simulink model "Switched_Reluctance_Motor_12bar8_config"  (R2021a)
settings: Solver=VariableStepAuto  StartTime=0.0  StopTime=1  FixedStep=1  MaxStep=1e-6  RelTol=1e-6
values from neighbouring files (symbols this model uses):
  angleArray = [0 0.5 1 1.5 2 2.5 3 3.5 4 4.5 5 5.5 ... (720 elements, 720x1)]    [matlab.mat]
  currentArray = [0 0.5 1 1.5 2 2.5 3 3.5 4 4.5 5 5.5 ... (51 elements, 51x1)]    [matlab.mat]
  fluxdiv = [0 4.83333e-05 9.66666e-05 0.000145 0.000193333 0.000241667 0.00029 0.000338333 0.000386666 0.000435 0.000483333 0.000531666 ... (720 elements, 720x1)]    [matlab.mat]
undefined symbols (not defined in the file or in its folder): iLUT, torqueMatrix
libraries: simulink x3, hdlsllib x1
settings Model: Creator=ADMIN  LastModifiedBy=Anirudh Chidambaram
settings SolverCC: AlgebraicLoopSolver=LineSearch
settings DataIOCC: SaveState=on
settings OptimizationCC: DefaultParameterBehavior=Inlined  EnhancedBackFolding=on  PassReuseOutputArgsAs=Individual arguments  ZeroExternalMemoryAtStartup=off  ZeroInternalMemoryAtStartup=off  OptimizeBlockOrder=speed  DifferentSizesBufferReuse=on  OptimizationCustomize=off  EfficientTunableParamExpr=on
settings DebuggingCC: AlgebraicLoopMsg=none  ParameterOverflowMsg=warning  ParameterTunabilityLossMsg=error  SFMachineParentedDataDiag=warning
settings SFSimCC: MATLABDynamicMemAlloc=off
settings RTWCC: SystemTargetFile=ert.tlc  TemplateMakefile=ert_default_tmf
settings CodeAppCC: ForceParamTrailComments=on  IgnoreCustomStorageClasses=off  OperatorAnnotations=on  SimulinkDataObjDesc=on  SFDataObjDesc=on  InsertBlockDesc=on
settings ERTTargetCC: TargetLangStandard=C99 (ISO)  GenerateSampleERTMain=on  InlinedParameterPlacement=NonHierarchical  ERTCustomFileTemplate=example_file_process.tlc

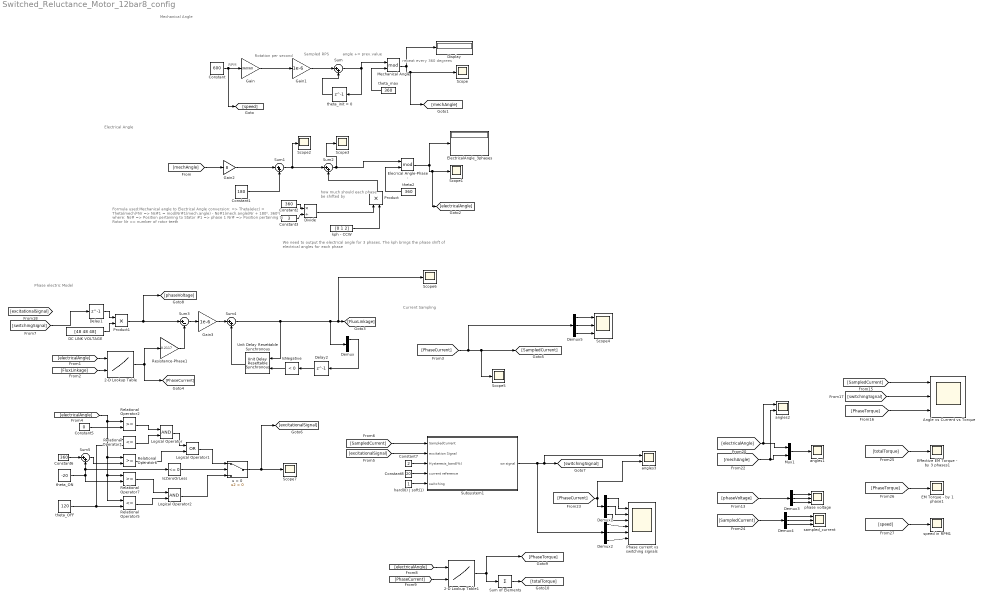
== system Switched_Reluctance_Motor_12bar8_config ==
  note: how much should each phase be shifted by
  note: repeat every 360 degrees
  note: angle += prev.value
  note: Sampled RPS
  note: Rotation per second
  note: RPM
  note: Electrical Angle
  note: Mechanical Angle
  note: Current Sampling
  note: Phase electric Model
  note: We need to output the electrical angle for 3 phases,
      | The kph brings the phase shift of electrical angles for each phase
  note: Formula used:Mechanical angle to Electrical Angle conversion:
      | => Theta(elec) = Theta(mech)*Nr
      |
      | => Ns#1 = mod(Nr#1(mech.angle) - Ns#1(mech.angle)Nr + 180⁰, 360⁰)
      | where:
      | Ns# => Position pertaining to Stator
      | #1	 => phase 1
      | Nr# => Position pertaining to Rotor
      | Nr	 => number of rotor teeth
  2-D Lookup Table : Lookup_n-D  BreakpointsForDimension1=angleArray  BreakpointsForDimension2=fluxdiv  Table=iLUT  InternalRulePriority=Speed  RndMeth=Simplest  InputSameDT=on
      settings: InputPortMap=u0,u1
  2-D Lookup Table1 : Lookup_n-D  BreakpointsForDimension1=angleArray  BreakpointsForDimension2=currentArray  Table=torqueMatrix  InternalRulePriority=Speed  RndMeth=Simplest  InputSameDT=on
      settings: InputPortMap=u0,u1
  Angle vs Current vs Torque : Scope  NumInputPorts=3
  Constant : Constant  Value=600  SampleTime=1e-6
  Constant1 : Constant  Value=180  SampleTime=1e-6
  Constant2 : Constant  Value=360  SampleTime=1e-6
  Constant3 : Constant  Value=3  SampleTime=1e-6
  Constant5 : Constant  Value=0
  Constant6 : Constant  Value=360
  Constant7 : Constant  Value=2
  Constant8 : Constant  Value=20
  DC LINK VOLTAGE : Constant  Value=[48 48 48]
  Delay1 : Delay  DelayLength=1
  Delay2 : Delay  DelayLength=1
  Demux{,1..5} (6 alike) : Demux  Outputs=3
  Display : Display
  Divide : Product  Inputs=*/
  EM Torque - by 1 phase1 : Scope
  Effective EM Torque - by 3 phases1 : Scope
  Elecrical Angle-Phase: : Math  Operator=mod  SaturateOnIntegerOverflow=on
  ElectricalAngle_3phases : Display
  Gain : Gain  Gain=360/60
  Gain1 : Gain  Gain=1e-6
  Gain2 : Gain  Gain=8
  Gain3 : Gain  Gain=1e-6
  IsNegative : simulink/Logic and Bit Operations/Compare To Zero  relop=<  OutDataTypeStr=boolean
  IsZeroOrLess : simulink/Logic and Bit Operations/Compare To Zero  relop=<=  OutDataTypeStr=boolean
  Logical Operator : Logic  AllPortsSameDT=off  OutDataTypeStr=boolean
  Logical Operator1 : Logic  Operator=OR  AllPortsSameDT=off  OutDataTypeStr=boolean
  Logical Operator2 : Logic  AllPortsSameDT=off  OutDataTypeStr=boolean
  Mechanical Angle : Math  Operator=mod  SaturateOnIntegerOverflow=on
  Mux1 : Mux  Inputs=2
  Phase current vs switching signals : Scope  NumInputPorts=6
  Product : Product
  Product1 : Product
  Relational Operator1 : RelationalOperator  Operator=<=  OutDataTypeStr=boolean  RndMeth=Simplest
  Relational Operator2 : RelationalOperator  OutDataTypeStr=boolean  RndMeth=Simplest
  Relational Operator5 : RelationalOperator  Operator=<=  OutDataTypeStr=boolean  RndMeth=Simplest
  Relational Operator6 : RelationalOperator  OutDataTypeStr=boolean  RndMeth=Simplest
  Relational Operator7 : RelationalOperator  OutDataTypeStr=boolean  RndMeth=Simplest
  Resistance-Phase1 : Gain  Gain=0.2117
  Scope{,1..3,5..7} (7 alike) : Scope
  Scope4 : Scope  NumInputPorts=3
  Subsystem1 : Subsystem
  Sum{,1..2,4..5} (5 alike) : Sum  Inputs=|++
  Sum of Elements : Sum  Inputs=+
  Sum3 : Sum  Inputs=|+-  RndMeth=Round
  Unit Delay Resettable Synchronous : hdlsllib/Discrete/Unit Delay Resettable Synchronous  InitialCondition=0.0  SampleTime=-1
      settings: SourceProductBaseCode=SL
  angles1 : Scope
  angles2 : Scope  NumInputPorts=2
  angles3 : Scope  NumInputPorts=2
  hard(0) | soft(1) : Constant
  kph - CCW : Constant  Value=[0 1 2]  SampleTime=1e-6
  phase voltage : Scope  NumInputPorts=3
  sampled_current : Scope  NumInputPorts=3
  speed in RPM1 : Scope
  theta2 : Constant  Value=360  SampleTime=1e-6
  theta_OFF : Constant  Value=120
  theta_ON : Constant  Value=-20
  theta_init = 0 : Delay  DelayLength=1  InitialCondition=0
  theta_max : Constant  Value=360  SampleTime=1e-6
  u > 0 : Switch  Criteria=u2 > Threshold
  wires:
  Mechanical Angle/1 -> [mechAngle], Scope/1, Display/1
  Constant/1 -> [speed], Gain/1
  theta_max/1 -> Mechanical Angle/2
  Gain1/1 -> Sum/1
  Sum/1 -> theta_init = 0/1, Mechanical Angle/1
  theta_init = 0/1 -> Sum/2
  Gain/1 -> Gain1/1
  Constant1/1 -> Sum1/2
  Gain2/1 -> Sum1/1
  Sum1/1 -> Scope2/1, Sum2/1
  Constant2/1 -> Divide/1
  Constant3/1 -> Divide/2
  Divide/1 -> Product/1
  kph - CCW/1 -> Product/2
  Product/1 -> Sum2/2
  Sum2/1 -> Scope3/1, Elecrical Angle-Phase:/1
  theta2/1 -> Elecrical Angle-Phase:/2
  Elecrical Angle-Phase:/1 -> [electricalAngle], Scope1/1, ElectricalAngle_3phases/1
  [mechAngle] -> Gain2/1
  Product1/1 -> [phaseVoltage], Sum3/1
  Sum3/1 -> Gain3/1
  Gain3/1 -> Sum4/1
  Resistance-Phase1/1 -> Sum3/2
  [FluxLinkage] -> 2-D Lookup Table/2
  2-D Lookup Table/1 -> [PhaseCurrent], Resistance-Phase1/1
  Delay2/1 -> IsNegative/1
  IsNegative/1 -> Unit Delay Resettable Synchronous/2
  Unit Delay Resettable Synchronous/1 -> Sum4/2
  Constant5/1 -> Relational Operator2/2
  [electricalAngle] -> Relational Operator5/1, Relational Operator7/1, Relational Operator6/1, Relational Operator1/1, Relational Operator2/1
  theta_ON/1 -> IsZeroOrLess/1, Sum5/2, Relational Operator7/2
  theta_OFF/1 -> Relational Operator1/2, Relational Operator5/2
  Constant6/1 -> Sum5/1
  Sum5/1 -> Relational Operator6/2
  Relational Operator1/1 -> Logical Operator/2
  Relational Operator2/1 -> Logical Operator/1
  Logical Operator/1 -> Logical Operator1/1
  Relational Operator6/1 -> Logical Operator1/2
  Relational Operator7/1 -> Logical Operator2/1
  Relational Operator5/1 -> Logical Operator2/2
  Logical Operator2/1 -> u > 0/3
  IsZeroOrLess/1 -> u > 0/2
  Logical Operator1/1 -> u > 0/1
  u > 0/1 -> Scope7/1, [excitationalSignal]
  [excitationalSignal] -> Subsystem1/2(excitation Signal)
  [SampledCurrent] -> Subsystem1/1(SampledCurrent)
  Constant8/1 -> Subsystem1/4(current reference)
  Constant7/1 -> Subsystem1/3(Hysteresis_band(%))
  hard(0) | soft(1)/1 -> Subsystem1/5(switching)
  Subsystem1/1(sw signal) -> Demux2/1, angles3/1, [switchingSignal]
  Delay1/1 -> Product1/1
  DC LINK VOLTAGE/1 -> Product1/2
  [electricalAngle] -> 2-D Lookup Table/1
  [electricalAngle] -> 2-D Lookup Table1/1
  [PhaseCurrent] -> 2-D Lookup Table1/2
  2-D Lookup Table1/1 -> [PhaseTorque], Sum of Elements/1
  Sum of Elements/1 -> [totalTorque]
  Sum4/1 -> Demux/1, Scope6/1, [FluxLinkage], Unit Delay Resettable Synchronous/1
  [SampledCurrent] -> Demux4/1
  [PhaseTorque] -> EM Torque - by 1 phase1/1
  [speed] -> speed in RPM1/1
  [electricalAngle] -> angles2/1, Mux1/1
  Mux1/1 -> angles1/1
  [totalTorque] -> Effective EM Torque - by 3 phases1/1
  [mechAngle] -> angles2/2, Mux1/2
  [PhaseCurrent] -> angles3/2, Demux1/1
  Demux/1 -> Delay2/1
  Demux1/1 -> Phase current vs switching signals/1
  Demux1/2 -> Phase current vs switching signals/2
  Demux1/3 -> Phase current vs switching signals/3
  Demux2/1 -> Phase current vs switching signals/4
  Demux2/2 -> Phase current vs switching signals/5
  Demux2/3 -> Phase current vs switching signals/6
  [phaseVoltage] -> Demux3/1
  Demux3/1 -> phase voltage/1
  Demux3/2 -> phase voltage/2
  Demux3/3 -> phase voltage/3
  Demux4/1 -> sampled_current/1
  Demux4/2 -> sampled_current/2
  Demux4/3 -> sampled_current/3
  [PhaseCurrent] -> Scope5/1, [SampledCurrent], Demux5/1
  Demux5/1 -> Scope4/1
  Demux5/2 -> Scope4/2
  Demux5/3 -> Scope4/3
  [SampledCurrent] -> Angle vs Current vs Torque/1
  [switchingSignal] -> Angle vs Current vs Torque/2
  [PhaseTorque] -> Angle vs Current vs Torque/3
  [switchingSignal] -> Delay1/1

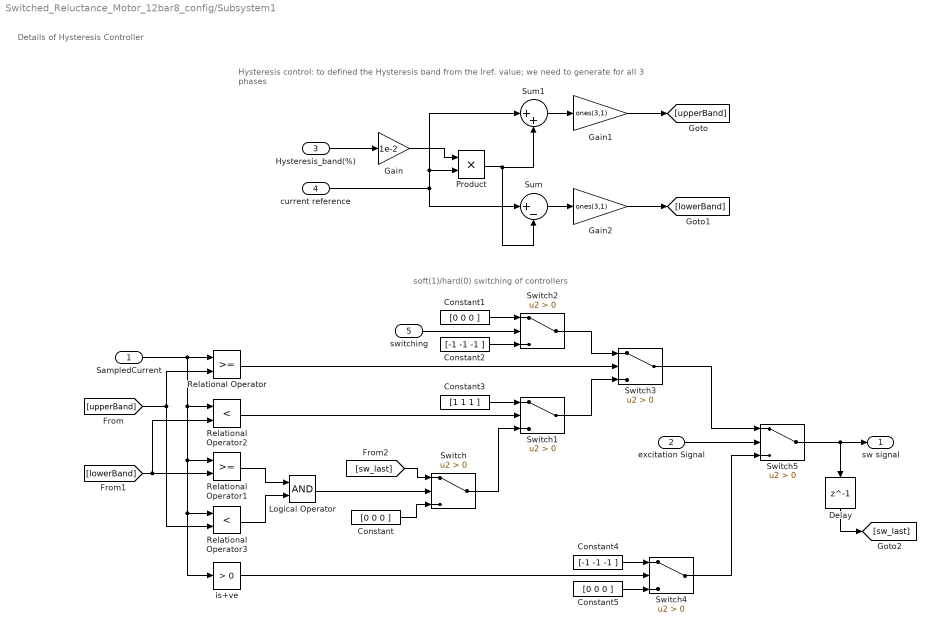
== system Switched_Reluctance_Motor_12bar8_config/Subsystem1 ==
  note: soft(1)/hard(0) switching of controllers
  note: Details of Hysteresis Controller
  note: Hysteresis control: to defined the Hysteresis band from the Iref. value; we need to generate for all 3 phases
  SampledCurrent : Inport
  excitation Signal : Inport  Port=2
  Hysteresis_band(%) : Inport  Port=3
  current reference : Inport  Port=4
  switching : Inport  Port=5
  Constant : Constant  Value=[0 0 0 ]
  Constant1 : Constant  Value=[0 0 0 ]
  Constant2 : Constant  Value=[-1 -1 -1 ]
  Constant3 : Constant  Value=[1 1 1 ]
  Constant4 : Constant  Value=[-1 -1 -1 ]
  Constant5 : Constant  Value=[0 0 0 ]
  Delay : Delay  DelayLength=1
  Gain : Gain  Gain=1e-2
  Gain1 : Gain  Gain=ones(3,1)
  Gain2 : Gain  Gain=ones(3,1)
  Logical Operator : Logic  AllPortsSameDT=off  OutDataTypeStr=boolean
  Product : Product
  Relational Operator : RelationalOperator  OutDataTypeStr=boolean  RndMeth=Simplest
  Relational Operator1 : RelationalOperator  OutDataTypeStr=boolean  RndMeth=Simplest
  Relational Operator2 : RelationalOperator  Operator=<  OutDataTypeStr=boolean  RndMeth=Simplest
  Relational Operator3 : RelationalOperator  Operator=<  OutDataTypeStr=boolean  RndMeth=Simplest
  Sum : Sum  Inputs=|+-
  Sum1 : Sum  Inputs=|++
  Switch{,1..5} (6 alike) : Switch  Criteria=u2 > Threshold
  is+ve : simulink/Logic and Bit Operations/Compare To Zero  relop=>  OutDataTypeStr=boolean
  sw signal : Outport
  wires:
  Gain/1 -> Product/1
  Hysteresis_band(%)/1 -> Gain/1
  current reference/1 -> Product/2, Sum1/1, Sum/1
  Product/1 -> Sum1/2, Sum/2
  Sum/1 -> Gain2/1
  Sum1/1 -> Gain1/1
  Gain1/1 -> [upperBand]
  Gain2/1 -> [lowerBand]
  [upperBand] -> Relational Operator/2, Relational Operator3/2
  [lowerBand] -> Relational Operator1/2, Relational Operator2/2
  SampledCurrent/1 -> Relational Operator/1, is+ve/1, Relational Operator3/1, Relational Operator1/1, Relational Operator2/1
  Relational Operator1/1 -> Logical Operator/1
  Relational Operator3/1 -> Logical Operator/2
  Relational Operator/1 -> Switch3/2
  Relational Operator2/1 -> Switch1/2
  [sw_last] -> Switch/1
  Logical Operator/1 -> Switch/2
  Constant/1 -> Switch/3
  switching/1 -> Switch2/2
  Constant1/1 -> Switch2/1
  Constant2/1 -> Switch2/3
  Switch2/1 -> Switch3/1
  Switch1/1 -> Switch3/3
  Constant3/1 -> Switch1/1
  Switch/1 -> Switch1/3
  is+ve/1 -> Switch4/2
  Constant4/1 -> Switch4/1
  Constant5/1 -> Switch4/3
  excitation Signal/1 -> Switch5/2
  Switch3/1 -> Switch5/1
  Switch4/1 -> Switch5/3
  Switch5/1 -> Delay/1, sw signal/1
  Delay/1 -> [sw_last]
